simulink model "Simulation"  (R2019b)
settings: Solver=VariableStepAuto  StartTime=0.0  StopTime=tmax  RelTol=1e-3
values from neighbouring files (symbols this model uses):
  BPden = [1 alpha]    [RunSimulation.m]    (also in RunTest.m)
  BPnum = [0.3 alpha]    [RunSimulation.m]    (also in RunTest.m)
  c = 250    [RunSimulation.m]    (also in RunTest.m)
  efficiency = 0.95    [RunSimulation.m]
  Fb = -1*m    (= -90000)    [RunSimulation.m]
  l = 18    [RunSimulation.m]    (also in RunTest.m)
  m = 90000    [RunSimulation.m]
  p0 = 0    [RunSimulation.m]    (also in RunTest.m)
  Pres = 0/1000*[5.7/771 0 1.6]    [RunSimulation.m]    (also in RunTest.m)
  RBD = 5    [RunSimulation.m]    (also in RunTest.m)
  tl = .1    (= 0.1)    [RunSimulation.m]    (also in RunTest.m)
  trackgradient = 0    [RunSimulation.m]    (also in RunTest.m)
  trainpower = m    (= 90000)    [RunSimulation.m]
  v0 = 100/3.6    (= 27.7777777778)    [RunSimulation.m]
  VBD = 3.5    [RunSimulation.m]    (also in RunTest.m)
libraries: simulink x11
(part 2 of 5)

== system Simulation/Subsystem1/Wagon model1 ==
  note: $F=F_a-F_{res}$
  note: $s(t)=v_{0}\cdot t-{1 \over 2}\cdot a\cdot t^{2}$
  note: $F=m\cdot a$ $a={F \over m}$
  p_BP : Inport
  In1 : Inport  Port=2
  Abs : Abs
  Add : Sum
  Clock : Clock
  Dead Zone : DeadZone  LowerValue=-0.001  UpperValue=0.001  SaturateOnIntegerOverflow=on
  Divide : Product  Inputs=*/
  Gain : Gain  Gain=-1/(RBD-VBD)
  Gain1 : Gain  Gain=Fb
  Gain2 : Gain  Gain=v0
  Gain3 : Gain  Gain=0.5
  Gravity : Gain  Gain=9.81
  Math Function : Math  Operator=square  SignedPower=off  SaturateOnIntegerOverflow=on
  Product : Product
  Product1 : Product
  Rate Limiter : RateLimiter  RisingSlewLimit=1/tf  FallingSlewLimit=-1/tl  SampleTimeMode=inherited
  Saturation : Saturate  UpperLimit=1  LowerLimit=0
  Strahl formula : Polyval  Coefs=Pres
  Subtract : Sum
  Sum1 : Sum  Inputs=|+-
  Transfer Fcn : TransferFcn  Numerator=BPnum  Denominator=BPden
  Transport Delay : TransportDelay  DelayTime=l/c  InitialOutput=p0
  efficiency : Gain  Gain=efficiency
  filter out going backwards : Saturate  UpperLimit=inf  LowerLimit=0
  mass : Constant  Value=m
  track gradient : Bias  Bias=9.81*sin(trackgradient)
  v = v0 + a * t : Integrator  InitialCondition=v0
  Fres : Outport  VectorParamsAs1DForOutWhenUnconnected=off
  p_BP_out : Outport  Port=2  VectorParamsAs1DForOutWhenUnconnected=off
  "v " : Outport  Port=3
  ares : Outport  Port=4
  st : Outport  Port=5
  wires:
  Strahl formula/1 -> Gravity/1
  Abs/1 -> "v "/1, Strahl formula/1
  Gravity/1 -> Product/2
  Product/1 -> Sum1/2  "Fw"
  v = v0 + a * t/1 -> Abs/1  "v"
  mass/1 -> Product/1, Divide/2
  Divide/1 -> track gradient/1  "a"
  p_BP/1 -> Transport Delay/1, Dead Zone/1
  Gain/1 -> Saturation/1
  Gain1/1 -> efficiency/1
  Saturation/1 -> Rate Limiter/1
  Rate Limiter/1 -> Gain1/1
  Transfer Fcn/1 -> p_BP_out/1
  Transport Delay/1 -> Transfer Fcn/1
  efficiency/1 -> Sum1/1
  track gradient/1 -> ares/1, Product1/2, v = v0 + a * t/1  "ares"
  Clock/1 -> Math Function/1, Gain2/1
  Math Function/1 -> Product1/1
  Product1/1 -> Gain3/1
  Subtract/1 -> filter out going backwards/1
  Gain3/1 -> Subtract/1
  Gain2/1 -> Subtract/2
  filter out going backwards/1 -> st/1
  Dead Zone/1 -> Gain/1
  In1/1 -> Add/1  "Fa"
  Sum1/1 -> Add/2  "Fres"
  Add/1 -> Fres/1, Divide/1  "F"

== system Simulation/Subsystem1/Wagon model2 ==
  note: $F=F_a-F_{res}$
  note: $s(t)=v_{0}\cdot t-{1 \over 2}\cdot a\cdot t^{2}$
  note: $F=m\cdot a$ $a={F \over m}$
  p_BP : Inport
  In1 : Inport  Port=2
  Abs : Abs
  Add : Sum
  Clock : Clock
  Dead Zone : DeadZone  LowerValue=-0.001  UpperValue=0.001  SaturateOnIntegerOverflow=on
  Divide : Product  Inputs=*/
  Gain : Gain  Gain=-1/(RBD-VBD)
  Gain1 : Gain  Gain=Fb
  Gain2 : Gain  Gain=v0
  Gain3 : Gain  Gain=0.5
  Gravity : Gain  Gain=9.81
  Math Function : Math  Operator=square  SignedPower=off  SaturateOnIntegerOverflow=on
  Product : Product
  Product1 : Product
  Rate Limiter : RateLimiter  RisingSlewLimit=1/tf  FallingSlewLimit=-1/tl  SampleTimeMode=inherited
  Saturation : Saturate  UpperLimit=1  LowerLimit=0
  Strahl formula : Polyval  Coefs=Pres
  Subtract : Sum
  Sum1 : Sum  Inputs=|+-
  Transfer Fcn : TransferFcn  Numerator=BPnum  Denominator=BPden
  Transport Delay : TransportDelay  DelayTime=l/c  InitialOutput=p0
  efficiency : Gain  Gain=efficiency
  filter out going backwards : Saturate  UpperLimit=inf  LowerLimit=0
  mass : Constant  Value=m
  track gradient : Bias  Bias=9.81*sin(trackgradient)
  v = v0 + a * t : Integrator  InitialCondition=v0
  Fres : Outport  VectorParamsAs1DForOutWhenUnconnected=off
  p_BP_out : Outport  Port=2  VectorParamsAs1DForOutWhenUnconnected=off
  "v " : Outport  Port=3
  ares : Outport  Port=4
  st : Outport  Port=5
  wires:
  Strahl formula/1 -> Gravity/1
  Abs/1 -> "v "/1, Strahl formula/1
  Gravity/1 -> Product/2
  Product/1 -> Sum1/2  "Fw"
  v = v0 + a * t/1 -> Abs/1  "v"
  mass/1 -> Product/1, Divide/2
  Divide/1 -> track gradient/1  "a"
  p_BP/1 -> Transport Delay/1, Dead Zone/1
  Gain/1 -> Saturation/1
  Gain1/1 -> efficiency/1
  Saturation/1 -> Rate Limiter/1
  Rate Limiter/1 -> Gain1/1
  Transfer Fcn/1 -> p_BP_out/1
  Transport Delay/1 -> Transfer Fcn/1
  efficiency/1 -> Sum1/1
  track gradient/1 -> ares/1, Product1/2, v = v0 + a * t/1  "ares"
  Clock/1 -> Math Function/1, Gain2/1
  Math Function/1 -> Product1/1
  Product1/1 -> Gain3/1
  Subtract/1 -> filter out going backwards/1
  Gain3/1 -> Subtract/1
  Gain2/1 -> Subtract/2
  filter out going backwards/1 -> st/1
  Dead Zone/1 -> Gain/1
  In1/1 -> Add/1  "Fa"
  Sum1/1 -> Add/2  "Fres"
  Add/1 -> Fres/1, Divide/1  "F"

== system Simulation/Subsystem1/Wagon model3 ==
  note: $F=F_a-F_{res}$
  note: $s(t)=v_{0}\cdot t-{1 \over 2}\cdot a\cdot t^{2}$
  note: $F=m\cdot a$ $a={F \over m}$
  p_BP : Inport
  In1 : Inport  Port=2
  Abs : Abs
  Add : Sum
  Clock : Clock
  Dead Zone : DeadZone  LowerValue=-0.001  UpperValue=0.001  SaturateOnIntegerOverflow=on
  Divide : Product  Inputs=*/
  Gain : Gain  Gain=-1/(RBD-VBD)
  Gain1 : Gain  Gain=Fb
  Gain2 : Gain  Gain=v0
  Gain3 : Gain  Gain=0.5
  Gravity : Gain  Gain=9.81
  Math Function : Math  Operator=square  SignedPower=off  SaturateOnIntegerOverflow=on
  Product : Product
  Product1 : Product
  Rate Limiter : RateLimiter  RisingSlewLimit=1/tf  FallingSlewLimit=-1/tl  SampleTimeMode=inherited
  Saturation : Saturate  UpperLimit=1  LowerLimit=0
  Strahl formula : Polyval  Coefs=Pres
  Subtract : Sum
  Sum1 : Sum  Inputs=|+-
  Transfer Fcn : TransferFcn  Numerator=BPnum  Denominator=BPden
  Transport Delay : TransportDelay  DelayTime=l/c  InitialOutput=p0
  efficiency : Gain  Gain=efficiency
  filter out going backwards : Saturate  UpperLimit=inf  LowerLimit=0
  mass : Constant  Value=m
  track gradient : Bias  Bias=9.81*sin(trackgradient)
  v = v0 + a * t : Integrator  InitialCondition=v0
  Fres : Outport  VectorParamsAs1DForOutWhenUnconnected=off
  p_BP_out : Outport  Port=2  VectorParamsAs1DForOutWhenUnconnected=off
  "v " : Outport  Port=3
  ares : Outport  Port=4
  st : Outport  Port=5
  wires:
  Strahl formula/1 -> Gravity/1
  Abs/1 -> "v "/1, Strahl formula/1
  Gravity/1 -> Product/2
  Product/1 -> Sum1/2  "Fw"
  v = v0 + a * t/1 -> Abs/1  "v"
  mass/1 -> Product/1, Divide/2
  Divide/1 -> track gradient/1  "a"
  p_BP/1 -> Transport Delay/1, Dead Zone/1
  Gain/1 -> Saturation/1
  Gain1/1 -> efficiency/1
  Saturation/1 -> Rate Limiter/1
  Rate Limiter/1 -> Gain1/1
  Transfer Fcn/1 -> p_BP_out/1
  Transport Delay/1 -> Transfer Fcn/1
  efficiency/1 -> Sum1/1
  track gradient/1 -> ares/1, Product1/2, v = v0 + a * t/1  "ares"
  Clock/1 -> Math Function/1, Gain2/1
  Math Function/1 -> Product1/1
  Product1/1 -> Gain3/1
  Subtract/1 -> filter out going backwards/1
  Gain3/1 -> Subtract/1
  Gain2/1 -> Subtract/2
  filter out going backwards/1 -> st/1
  Dead Zone/1 -> Gain/1
  In1/1 -> Add/1  "Fa"
  Sum1/1 -> Add/2  "Fres"
  Add/1 -> Fres/1, Divide/1  "F"

== system Simulation/Subsystem1/Wagon model4 ==
  note: $F=F_a-F_{res}$
  note: $s(t)=v_{0}\cdot t-{1 \over 2}\cdot a\cdot t^{2}$
  note: $F=m\cdot a$ $a={F \over m}$
  p_BP : Inport
  In1 : Inport  Port=2
  Abs : Abs
  Add : Sum
  Clock : Clock
  Dead Zone : DeadZone  LowerValue=-0.001  UpperValue=0.001  SaturateOnIntegerOverflow=on
  Divide : Product  Inputs=*/
  Gain : Gain  Gain=-1/(RBD-VBD)
  Gain1 : Gain  Gain=Fb
  Gain2 : Gain  Gain=v0
  Gain3 : Gain  Gain=0.5
  Gravity : Gain  Gain=9.81
  Math Function : Math  Operator=square  SignedPower=off  SaturateOnIntegerOverflow=on
  Product : Product
  Product1 : Product
  Rate Limiter : RateLimiter  RisingSlewLimit=1/tf  FallingSlewLimit=-1/tl  SampleTimeMode=inherited
  Saturation : Saturate  UpperLimit=1  LowerLimit=0
  Strahl formula : Polyval  Coefs=Pres
  Subtract : Sum
  Sum1 : Sum  Inputs=|+-
  Transfer Fcn : TransferFcn  Numerator=BPnum  Denominator=BPden
  Transport Delay : TransportDelay  DelayTime=l/c  InitialOutput=p0
  efficiency : Gain  Gain=efficiency
  filter out going backwards : Saturate  UpperLimit=inf  LowerLimit=0
  mass : Constant  Value=m
  track gradient : Bias  Bias=9.81*sin(trackgradient)
  v = v0 + a * t : Integrator  InitialCondition=v0
  Fres : Outport  VectorParamsAs1DForOutWhenUnconnected=off
  p_BP_out : Outport  Port=2  VectorParamsAs1DForOutWhenUnconnected=off
  "v " : Outport  Port=3
  ares : Outport  Port=4
  st : Outport  Port=5
  wires:
  Strahl formula/1 -> Gravity/1
  Abs/1 -> "v "/1, Strahl formula/1
  Gravity/1 -> Product/2
  Product/1 -> Sum1/2  "Fw"
  v = v0 + a * t/1 -> Abs/1  "v"
  mass/1 -> Product/1, Divide/2
  Divide/1 -> track gradient/1  "a"
  p_BP/1 -> Transport Delay/1, Dead Zone/1
  Gain/1 -> Saturation/1
  Gain1/1 -> efficiency/1
  Saturation/1 -> Rate Limiter/1
  Rate Limiter/1 -> Gain1/1
  Transfer Fcn/1 -> p_BP_out/1
  Transport Delay/1 -> Transfer Fcn/1
  efficiency/1 -> Sum1/1
  track gradient/1 -> ares/1, Product1/2, v = v0 + a * t/1  "ares"
  Clock/1 -> Math Function/1, Gain2/1
  Math Function/1 -> Product1/1
  Product1/1 -> Gain3/1
  Subtract/1 -> filter out going backwards/1
  Gain3/1 -> Subtract/1
  Gain2/1 -> Subtract/2
  filter out going backwards/1 -> st/1
  Dead Zone/1 -> Gain/1
  In1/1 -> Add/1  "Fa"
  Sum1/1 -> Add/2  "Fres"
  Add/1 -> Fres/1, Divide/1  "F"

== system Simulation/Subsystem10/Wagon model ==
  note: F = m * a
      | a = F / m
  p_BP : Inport
  Abs : Abs
  Constant : Constant  Value=m
  Divide : Product  Inputs=*/
  Gain : Gain  Gain=-1/(RBD-VBD)
  Gain1 : Gain  Gain=Fb
  Gravity : Gain  Gain=9.81
  Product : Product
  Rate Limiter : RateLimiter  RisingSlewLimit=1/tf  FallingSlewLimit=-1/tl  SampleTimeMode=inherited
  Saturation : Saturate  UpperLimit=1  LowerLimit=0
  Strahl formula : Polyval  Coefs=Pres
  Sum1 : Sum  Inputs=|+-
  Transfer Fcn : TransferFcn  Numerator=BPnum  Denominator=BPden
  Transport Delay : TransportDelay  DelayTime=l/c  InitialOutput=p0
  filter out negative velocity : Saturate  UpperLimit=inf  LowerLimit=0
  v = v0 + a * t : Integrator  InitialCondition=v0
  Fres : Outport  VectorParamsAs1DForOutWhenUnconnected=off
  p_BP_out : Outport  Port=2  VectorParamsAs1DForOutWhenUnconnected=off
  "v " : Outport  Port=3
  wires:
  Sum1/1 -> Fres/1, Divide/1  "Fres"
  Strahl formula/1 -> Gravity/1
  Abs/1 -> Strahl formula/1
  Gravity/1 -> Product/2
  Product/1 -> Sum1/2  "Fw"
  v = v0 + a * t/1 -> filter out negative velocity/1, Abs/1  "v"
  Constant/1 -> Product/1, Divide/2
  Divide/1 -> v = v0 + a * t/1  "a"
  p_BP/1 -> Transport Delay/1, Gain/1
  Gain/1 -> Saturation/1
  Gain1/1 -> Sum1/1
  Saturation/1 -> Rate Limiter/1
  Rate Limiter/1 -> Gain1/1
  Transfer Fcn/1 -> p_BP_out/1
  Transport Delay/1 -> Transfer Fcn/1
  filter out negative velocity/1 -> "v "/1

== system Simulation/Subsystem10/Wagon model1 ==
  p_BP : Inport
  Abs : Abs
  Constant : Constant  Value=m
  Divide : Product  Inputs=*/
  Gain : Gain  Gain=-1/(RBD-VBD)
  Gain1 : Gain  Gain=Fb
  Gravity : Gain  Gain=9.81
  Integrator : Integrator  InitialCondition=v0
  Product : Product
  Rate Limiter : RateLimiter  RisingSlewLimit=1/tf  FallingSlewLimit=-1/tl  SampleTimeMode=inherited
  Saturation : Saturate  UpperLimit=1  LowerLimit=0
  Strahl formula : Polyval  Coefs=Pres
  Sum1 : Sum  Inputs=|+-
  Transfer Fcn : TransferFcn  Numerator=BPnum  Denominator=BPden
  Transport Delay : TransportDelay  DelayTime=l/c  InitialOutput=p0
  filter out negative velocity : Saturate  UpperLimit=inf  LowerLimit=0
  Fres : Outport  VectorParamsAs1DForOutWhenUnconnected=off
  p_BP_out : Outport  Port=2  VectorParamsAs1DForOutWhenUnconnected=off
  "v " : Outport  Port=3
  wires:
  Sum1/1 -> Fres/1, Divide/1  "Fres"
  Strahl formula/1 -> Gravity/1
  Abs/1 -> Strahl formula/1
  Gravity/1 -> Product/2
  Product/1 -> Sum1/2  "Fw"
  Integrator/1 -> filter out negative velocity/1, Abs/1  "v"
  Constant/1 -> Product/1, Divide/2
  Divide/1 -> Integrator/1  "a"
  p_BP/1 -> Gain/1, Transport Delay/1
  Gain/1 -> Saturation/1
  Gain1/1 -> Sum1/1
  Saturation/1 -> Rate Limiter/1
  Rate Limiter/1 -> Gain1/1
  Transport Delay/1 -> Transfer Fcn/1
  Transfer Fcn/1 -> p_BP_out/1
  filter out negative velocity/1 -> "v "/1

== system Simulation/Subsystem10/Wagon model2 ==
  p_BP : Inport
  Abs : Abs
  Constant : Constant  Value=m
  Divide : Product  Inputs=*/
  Gain : Gain  Gain=-1/(RBD-VBD)
  Gain1 : Gain  Gain=Fb
  Gravity : Gain  Gain=9.81
  Integrator : Integrator  InitialCondition=v0
  Product : Product
  Rate Limiter : RateLimiter  RisingSlewLimit=1/tf  FallingSlewLimit=-1/tl  SampleTimeMode=inherited
  Saturation : Saturate  UpperLimit=1  LowerLimit=0
  Strahl formula : Polyval  Coefs=Pres
  Sum1 : Sum  Inputs=|+-
  Transfer Fcn : TransferFcn  Numerator=BPnum  Denominator=BPden
  Transport Delay : TransportDelay  DelayTime=l/c  InitialOutput=p0
  filter out negative velocity : Saturate  UpperLimit=inf  LowerLimit=0
  Fres : Outport  VectorParamsAs1DForOutWhenUnconnected=off
  p_BP_out : Outport  Port=2  VectorParamsAs1DForOutWhenUnconnected=off
  "v " : Outport  Port=3
  wires:
  Sum1/1 -> Fres/1, Divide/1  "Fres"
  Strahl formula/1 -> Gravity/1
  Abs/1 -> Strahl formula/1
  Gravity/1 -> Product/2
  Product/1 -> Sum1/2  "Fw"
  Constant/1 -> Product/1, Divide/2
  Divide/1 -> Integrator/1  "a"
  p_BP/1 -> Gain/1, Transport Delay/1
  Gain/1 -> Saturation/1
  Gain1/1 -> Sum1/1
  Saturation/1 -> Rate Limiter/1
  Rate Limiter/1 -> Gain1/1
  Transport Delay/1 -> Transfer Fcn/1
  Transfer Fcn/1 -> p_BP_out/1
  Integrator/1 -> filter out negative velocity/1, Abs/1  "v"
  filter out negative velocity/1 -> "v "/1

== system Simulation/Subsystem10/Wagon model3 ==
  p_BP : Inport
  Abs : Abs
  Constant : Constant  Value=m
  Divide : Product  Inputs=*/
  Gain : Gain  Gain=-1/(RBD-VBD)
  Gain1 : Gain  Gain=Fb
  Gravity : Gain  Gain=9.81
  Integrator : Integrator  InitialCondition=v0
  Product : Product
  Rate Limiter : RateLimiter  RisingSlewLimit=1/tf  FallingSlewLimit=-1/tl  SampleTimeMode=inherited
  Saturation : Saturate  UpperLimit=1  LowerLimit=0
  Strahl formula : Polyval  Coefs=Pres
  Sum1 : Sum  Inputs=|+-
  Transfer Fcn : TransferFcn  Numerator=BPnum  Denominator=BPden
  Transport Delay : TransportDelay  DelayTime=l/c  InitialOutput=p0
  filter out negative velocity : Saturate  UpperLimit=inf  LowerLimit=0
  Fres : Outport  VectorParamsAs1DForOutWhenUnconnected=off
  p_BP_out : Outport  Port=2  VectorParamsAs1DForOutWhenUnconnected=off
  "v " : Outport  Port=3
  wires:
  Sum1/1 -> Fres/1, Divide/1  "Fres"
  Strahl formula/1 -> Gravity/1
  Abs/1 -> Strahl formula/1
  Gravity/1 -> Product/2
  Product/1 -> Sum1/2  "Fw"
  Constant/1 -> Product/1, Divide/2
  Divide/1 -> Integrator/1  "a"
  p_BP/1 -> Gain/1, Transport Delay/1
  Gain/1 -> Saturation/1
  Gain1/1 -> Sum1/1
  Saturation/1 -> Rate Limiter/1
  Rate Limiter/1 -> Gain1/1
  Transport Delay/1 -> Transfer Fcn/1
  Transfer Fcn/1 -> p_BP_out/1
  Integrator/1 -> Abs/1, filter out negative velocity/1  "v"
  filter out negative velocity/1 -> "v "/1

== system Simulation/Subsystem10/Wagon model4 ==
  p_BP : Inport
  Abs : Abs
  Constant : Constant  Value=m
  Divide : Product  Inputs=*/
  Gain : Gain  Gain=-1/(RBD-VBD)
  Gain1 : Gain  Gain=Fb
  Gravity : Gain  Gain=9.81
  Integrator : Integrator  InitialCondition=v0
  Product : Product
  Rate Limiter : RateLimiter  RisingSlewLimit=1/tf  FallingSlewLimit=-1/tl  SampleTimeMode=inherited
  Saturation : Saturate  UpperLimit=1  LowerLimit=0
  Strahl formula : Polyval  Coefs=Pres
  Sum1 : Sum  Inputs=|+-
  Transfer Fcn : TransferFcn  Numerator=BPnum  Denominator=BPden
  Transport Delay : TransportDelay  DelayTime=l/c  InitialOutput=p0
  filter out negative velocity : Saturate  UpperLimit=inf  LowerLimit=0
  Fres : Outport  VectorParamsAs1DForOutWhenUnconnected=off
  p_BP_out : Outport  Port=2  VectorParamsAs1DForOutWhenUnconnected=off
  "v " : Outport  Port=3
  wires:
  Sum1/1 -> Fres/1, Divide/1  "Fres"
  Strahl formula/1 -> Gravity/1
  Abs/1 -> Strahl formula/1
  Gravity/1 -> Product/2
  Product/1 -> Sum1/2  "Fw"
  Integrator/1 -> filter out negative velocity/1, Abs/1  "v"
  Constant/1 -> Product/1, Divide/2
  Divide/1 -> Integrator/1  "a"
  p_BP/1 -> Gain/1, Transport Delay/1
  Gain/1 -> Saturation/1
  Gain1/1 -> Sum1/1
  Saturation/1 -> Rate Limiter/1
  Rate Limiter/1 -> Gain1/1
  Transfer Fcn/1 -> p_BP_out/1
  Transport Delay/1 -> Transfer Fcn/1
  filter out negative velocity/1 -> "v "/1

== system Simulation/Subsystem11/Wagon model ==
  note: F = m * a
      | a = F / m
  p_BP : Inport
  Abs : Abs
  Constant : Constant  Value=m
  Divide : Product  Inputs=*/
  Gain : Gain  Gain=-1/(RBD-VBD)
  Gain1 : Gain  Gain=Fb
  Gravity : Gain  Gain=9.81
  Product : Product
  Rate Limiter : RateLimiter  RisingSlewLimit=1/tf  FallingSlewLimit=-1/tl  SampleTimeMode=inherited
  Saturation : Saturate  UpperLimit=1  LowerLimit=0
  Strahl formula : Polyval  Coefs=Pres
  Sum1 : Sum  Inputs=|+-
  Transfer Fcn : TransferFcn  Numerator=BPnum  Denominator=BPden
  Transport Delay : TransportDelay  DelayTime=l/c  InitialOutput=p0
  filter out negative velocity : Saturate  UpperLimit=inf  LowerLimit=0
  v = v0 + a * t : Integrator  InitialCondition=v0
  Fres : Outport  VectorParamsAs1DForOutWhenUnconnected=off
  p_BP_out : Outport  Port=2  VectorParamsAs1DForOutWhenUnconnected=off
  "v " : Outport  Port=3
  wires:
  Sum1/1 -> Fres/1, Divide/1  "Fres"
  Strahl formula/1 -> Gravity/1
  Abs/1 -> Strahl formula/1
  Gravity/1 -> Product/2
  Product/1 -> Sum1/2  "Fw"
  v = v0 + a * t/1 -> filter out negative velocity/1, Abs/1  "v"
  Constant/1 -> Product/1, Divide/2
  Divide/1 -> v = v0 + a * t/1  "a"
  p_BP/1 -> Transport Delay/1, Gain/1
  Gain/1 -> Saturation/1
  Gain1/1 -> Sum1/1
  Saturation/1 -> Rate Limiter/1
  Rate Limiter/1 -> Gain1/1
  Transfer Fcn/1 -> p_BP_out/1
  Transport Delay/1 -> Transfer Fcn/1
  filter out negative velocity/1 -> "v "/1

== system Simulation/Subsystem11/Wagon model1 ==
  p_BP : Inport
  Abs : Abs
  Constant : Constant  Value=m
  Divide : Product  Inputs=*/
  Gain : Gain  Gain=-1/(RBD-VBD)
  Gain1 : Gain  Gain=Fb
  Gravity : Gain  Gain=9.81
  Integrator : Integrator  InitialCondition=v0
  Product : Product
  Rate Limiter : RateLimiter  RisingSlewLimit=1/tf  FallingSlewLimit=-1/tl  SampleTimeMode=inherited
  Saturation : Saturate  UpperLimit=1  LowerLimit=0
  Strahl formula : Polyval  Coefs=Pres
  Sum1 : Sum  Inputs=|+-
  Transfer Fcn : TransferFcn  Numerator=BPnum  Denominator=BPden
  Transport Delay : TransportDelay  DelayTime=l/c  InitialOutput=p0
  filter out negative velocity : Saturate  UpperLimit=inf  LowerLimit=0
  Fres : Outport  VectorParamsAs1DForOutWhenUnconnected=off
  p_BP_out : Outport  Port=2  VectorParamsAs1DForOutWhenUnconnected=off
  "v " : Outport  Port=3
  wires:
  Sum1/1 -> Fres/1, Divide/1  "Fres"
  Strahl formula/1 -> Gravity/1
  Abs/1 -> Strahl formula/1
  Gravity/1 -> Product/2
  Product/1 -> Sum1/2  "Fw"
  Integrator/1 -> filter out negative velocity/1, Abs/1  "v"
  Constant/1 -> Product/1, Divide/2
  Divide/1 -> Integrator/1  "a"
  p_BP/1 -> Gain/1, Transport Delay/1
  Gain/1 -> Saturation/1
  Gain1/1 -> Sum1/1
  Saturation/1 -> Rate Limiter/1
  Rate Limiter/1 -> Gain1/1
  Transport Delay/1 -> Transfer Fcn/1
  Transfer Fcn/1 -> p_BP_out/1
  filter out negative velocity/1 -> "v "/1

== system Simulation/Subsystem11/Wagon model2 ==
  p_BP : Inport
  Abs : Abs
  Constant : Constant  Value=m
  Divide : Product  Inputs=*/
  Gain : Gain  Gain=-1/(RBD-VBD)
  Gain1 : Gain  Gain=Fb
  Gravity : Gain  Gain=9.81
  Integrator : Integrator  InitialCondition=v0
  Product : Product
  Rate Limiter : RateLimiter  RisingSlewLimit=1/tf  FallingSlewLimit=-1/tl  SampleTimeMode=inherited
  Saturation : Saturate  UpperLimit=1  LowerLimit=0
  Strahl formula : Polyval  Coefs=Pres
  Sum1 : Sum  Inputs=|+-
  Transfer Fcn : TransferFcn  Numerator=BPnum  Denominator=BPden
  Transport Delay : TransportDelay  DelayTime=l/c  InitialOutput=p0
  filter out negative velocity : Saturate  UpperLimit=inf  LowerLimit=0
  Fres : Outport  VectorParamsAs1DForOutWhenUnconnected=off
  p_BP_out : Outport  Port=2  VectorParamsAs1DForOutWhenUnconnected=off
  "v " : Outport  Port=3
  wires:
  Sum1/1 -> Fres/1, Divide/1  "Fres"
  Strahl formula/1 -> Gravity/1
  Abs/1 -> Strahl formula/1
  Gravity/1 -> Product/2
  Product/1 -> Sum1/2  "Fw"
  Constant/1 -> Product/1, Divide/2
  Divide/1 -> Integrator/1  "a"
  p_BP/1 -> Gain/1, Transport Delay/1
  Gain/1 -> Saturation/1
  Gain1/1 -> Sum1/1
  Saturation/1 -> Rate Limiter/1
  Rate Limiter/1 -> Gain1/1
  Transport Delay/1 -> Transfer Fcn/1
  Transfer Fcn/1 -> p_BP_out/1
  Integrator/1 -> filter out negative velocity/1, Abs/1  "v"
  filter out negative velocity/1 -> "v "/1

== system Simulation/Subsystem11/Wagon model3 ==
  p_BP : Inport
  Abs : Abs
  Constant : Constant  Value=m
  Divide : Product  Inputs=*/
  Gain : Gain  Gain=-1/(RBD-VBD)
  Gain1 : Gain  Gain=Fb
  Gravity : Gain  Gain=9.81
  Integrator : Integrator  InitialCondition=v0
  Product : Product
  Rate Limiter : RateLimiter  RisingSlewLimit=1/tf  FallingSlewLimit=-1/tl  SampleTimeMode=inherited
  Saturation : Saturate  UpperLimit=1  LowerLimit=0
  Strahl formula : Polyval  Coefs=Pres
  Sum1 : Sum  Inputs=|+-
  Transfer Fcn : TransferFcn  Numerator=BPnum  Denominator=BPden
  Transport Delay : TransportDelay  DelayTime=l/c  InitialOutput=p0
  filter out negative velocity : Saturate  UpperLimit=inf  LowerLimit=0
  Fres : Outport  VectorParamsAs1DForOutWhenUnconnected=off
  p_BP_out : Outport  Port=2  VectorParamsAs1DForOutWhenUnconnected=off
  "v " : Outport  Port=3
  wires:
  Sum1/1 -> Fres/1, Divide/1  "Fres"
  Strahl formula/1 -> Gravity/1
  Abs/1 -> Strahl formula/1
  Gravity/1 -> Product/2
  Product/1 -> Sum1/2  "Fw"
  Constant/1 -> Product/1, Divide/2
  Divide/1 -> Integrator/1  "a"
  p_BP/1 -> Gain/1, Transport Delay/1
  Gain/1 -> Saturation/1
  Gain1/1 -> Sum1/1
  Saturation/1 -> Rate Limiter/1
  Rate Limiter/1 -> Gain1/1
  Transport Delay/1 -> Transfer Fcn/1
  Transfer Fcn/1 -> p_BP_out/1
  Integrator/1 -> Abs/1, filter out negative velocity/1  "v"
  filter out negative velocity/1 -> "v "/1

== system Simulation/Subsystem11/Wagon model4 ==
  p_BP : Inport
  Abs : Abs
  Constant : Constant  Value=m
  Divide : Product  Inputs=*/
  Gain : Gain  Gain=-1/(RBD-VBD)
  Gain1 : Gain  Gain=Fb
  Gravity : Gain  Gain=9.81
  Integrator : Integrator  InitialCondition=v0
  Product : Product
  Rate Limiter : RateLimiter  RisingSlewLimit=1/tf  FallingSlewLimit=-1/tl  SampleTimeMode=inherited
  Saturation : Saturate  UpperLimit=1  LowerLimit=0
  Strahl formula : Polyval  Coefs=Pres
  Sum1 : Sum  Inputs=|+-
  Transfer Fcn : TransferFcn  Numerator=BPnum  Denominator=BPden
  Transport Delay : TransportDelay  DelayTime=l/c  InitialOutput=p0
  filter out negative velocity : Saturate  UpperLimit=inf  LowerLimit=0
  Fres : Outport  VectorParamsAs1DForOutWhenUnconnected=off
  p_BP_out : Outport  Port=2  VectorParamsAs1DForOutWhenUnconnected=off
  "v " : Outport  Port=3
  wires:
  Sum1/1 -> Fres/1, Divide/1  "Fres"
  Strahl formula/1 -> Gravity/1
  Abs/1 -> Strahl formula/1
  Gravity/1 -> Product/2
  Product/1 -> Sum1/2  "Fw"
  Integrator/1 -> filter out negative velocity/1, Abs/1  "v"
  Constant/1 -> Product/1, Divide/2
  Divide/1 -> Integrator/1  "a"
  p_BP/1 -> Gain/1, Transport Delay/1
  Gain/1 -> Saturation/1
  Gain1/1 -> Sum1/1
  Saturation/1 -> Rate Limiter/1
  Rate Limiter/1 -> Gain1/1
  Transfer Fcn/1 -> p_BP_out/1
  Transport Delay/1 -> Transfer Fcn/1
  filter out negative velocity/1 -> "v "/1

== system Simulation/Subsystem12/Wagon model ==
  note: F = m * a
      | a = F / m
  p_BP : Inport
  Abs : Abs
  Constant : Constant  Value=m
  Divide : Product  Inputs=*/
  Gain : Gain  Gain=-1/(RBD-VBD)
  Gain1 : Gain  Gain=Fb
  Gravity : Gain  Gain=9.81
  Product : Product
  Rate Limiter : RateLimiter  RisingSlewLimit=1/tf  FallingSlewLimit=-1/tl  SampleTimeMode=inherited
  Saturation : Saturate  UpperLimit=1  LowerLimit=0
  Strahl formula : Polyval  Coefs=Pres
  Sum1 : Sum  Inputs=|+-
  Transfer Fcn : TransferFcn  Numerator=BPnum  Denominator=BPden
  Transport Delay : TransportDelay  DelayTime=l/c  InitialOutput=p0
  filter out negative velocity : Saturate  UpperLimit=inf  LowerLimit=0
  v = v0 + a * t : Integrator  InitialCondition=v0
  Fres : Outport  VectorParamsAs1DForOutWhenUnconnected=off
  p_BP_out : Outport  Port=2  VectorParamsAs1DForOutWhenUnconnected=off
  "v " : Outport  Port=3
  wires:
  Sum1/1 -> Fres/1, Divide/1  "Fres"
  Strahl formula/1 -> Gravity/1
  Abs/1 -> Strahl formula/1
  Gravity/1 -> Product/2
  Product/1 -> Sum1/2  "Fw"
  v = v0 + a * t/1 -> filter out negative velocity/1, Abs/1  "v"
  Constant/1 -> Product/1, Divide/2
  Divide/1 -> v = v0 + a * t/1  "a"
  p_BP/1 -> Transport Delay/1, Gain/1
  Gain/1 -> Saturation/1
  Gain1/1 -> Sum1/1
  Saturation/1 -> Rate Limiter/1
  Rate Limiter/1 -> Gain1/1
  Transfer Fcn/1 -> p_BP_out/1
  Transport Delay/1 -> Transfer Fcn/1
  filter out negative velocity/1 -> "v "/1

== system Simulation/Subsystem12/Wagon model1 ==
  p_BP : Inport
  Abs : Abs
  Constant : Constant  Value=m
  Divide : Product  Inputs=*/
  Gain : Gain  Gain=-1/(RBD-VBD)
  Gain1 : Gain  Gain=Fb
  Gravity : Gain  Gain=9.81
  Integrator : Integrator  InitialCondition=v0
  Product : Product
  Rate Limiter : RateLimiter  RisingSlewLimit=1/tf  FallingSlewLimit=-1/tl  SampleTimeMode=inherited
  Saturation : Saturate  UpperLimit=1  LowerLimit=0
  Strahl formula : Polyval  Coefs=Pres
  Sum1 : Sum  Inputs=|+-
  Transfer Fcn : TransferFcn  Numerator=BPnum  Denominator=BPden
  Transport Delay : TransportDelay  DelayTime=l/c  InitialOutput=p0
  filter out negative velocity : Saturate  UpperLimit=inf  LowerLimit=0
  Fres : Outport  VectorParamsAs1DForOutWhenUnconnected=off
  p_BP_out : Outport  Port=2  VectorParamsAs1DForOutWhenUnconnected=off
  "v " : Outport  Port=3
  wires:
  Sum1/1 -> Fres/1, Divide/1  "Fres"
  Strahl formula/1 -> Gravity/1
  Abs/1 -> Strahl formula/1
  Gravity/1 -> Product/2
  Product/1 -> Sum1/2  "Fw"
  Integrator/1 -> filter out negative velocity/1, Abs/1  "v"
  Constant/1 -> Product/1, Divide/2
  Divide/1 -> Integrator/1  "a"
  p_BP/1 -> Gain/1, Transport Delay/1
  Gain/1 -> Saturation/1
  Gain1/1 -> Sum1/1
  Saturation/1 -> Rate Limiter/1
  Rate Limiter/1 -> Gain1/1
  Transport Delay/1 -> Transfer Fcn/1
  Transfer Fcn/1 -> p_BP_out/1
  filter out negative velocity/1 -> "v "/1

== system Simulation/Subsystem12/Wagon model2 ==
  p_BP : Inport
  Abs : Abs
  Constant : Constant  Value=m
  Divide : Product  Inputs=*/
  Gain : Gain  Gain=-1/(RBD-VBD)
  Gain1 : Gain  Gain=Fb
  Gravity : Gain  Gain=9.81
  Integrator : Integrator  InitialCondition=v0
  Product : Product
  Rate Limiter : RateLimiter  RisingSlewLimit=1/tf  FallingSlewLimit=-1/tl  SampleTimeMode=inherited
  Saturation : Saturate  UpperLimit=1  LowerLimit=0
  Strahl formula : Polyval  Coefs=Pres
  Sum1 : Sum  Inputs=|+-
  Transfer Fcn : TransferFcn  Numerator=BPnum  Denominator=BPden
  Transport Delay : TransportDelay  DelayTime=l/c  InitialOutput=p0
  filter out negative velocity : Saturate  UpperLimit=inf  LowerLimit=0
  Fres : Outport  VectorParamsAs1DForOutWhenUnconnected=off
  p_BP_out : Outport  Port=2  VectorParamsAs1DForOutWhenUnconnected=off
  "v " : Outport  Port=3
  wires:
  Sum1/1 -> Fres/1, Divide/1  "Fres"
  Strahl formula/1 -> Gravity/1
  Abs/1 -> Strahl formula/1
  Gravity/1 -> Product/2
  Product/1 -> Sum1/2  "Fw"
  Constant/1 -> Product/1, Divide/2
  Divide/1 -> Integrator/1  "a"
  p_BP/1 -> Gain/1, Transport Delay/1
  Gain/1 -> Saturation/1
  Gain1/1 -> Sum1/1
  Saturation/1 -> Rate Limiter/1
  Rate Limiter/1 -> Gain1/1
  Transport Delay/1 -> Transfer Fcn/1
  Transfer Fcn/1 -> p_BP_out/1
  Integrator/1 -> filter out negative velocity/1, Abs/1  "v"
  filter out negative velocity/1 -> "v "/1

== system Simulation/Subsystem12/Wagon model3 ==
  p_BP : Inport
  Abs : Abs
  Constant : Constant  Value=m
  Divide : Product  Inputs=*/
  Gain : Gain  Gain=-1/(RBD-VBD)
  Gain1 : Gain  Gain=Fb
  Gravity : Gain  Gain=9.81
  Integrator : Integrator  InitialCondition=v0
  Product : Product
  Rate Limiter : RateLimiter  RisingSlewLimit=1/tf  FallingSlewLimit=-1/tl  SampleTimeMode=inherited
  Saturation : Saturate  UpperLimit=1  LowerLimit=0
  Strahl formula : Polyval  Coefs=Pres
  Sum1 : Sum  Inputs=|+-
  Transfer Fcn : TransferFcn  Numerator=BPnum  Denominator=BPden
  Transport Delay : TransportDelay  DelayTime=l/c  InitialOutput=p0
  filter out negative velocity : Saturate  UpperLimit=inf  LowerLimit=0
  Fres : Outport  VectorParamsAs1DForOutWhenUnconnected=off
  p_BP_out : Outport  Port=2  VectorParamsAs1DForOutWhenUnconnected=off
  "v " : Outport  Port=3
  wires:
  Sum1/1 -> Fres/1, Divide/1  "Fres"
  Strahl formula/1 -> Gravity/1
  Abs/1 -> Strahl formula/1
  Gravity/1 -> Product/2
  Product/1 -> Sum1/2  "Fw"
  Constant/1 -> Product/1, Divide/2
  Divide/1 -> Integrator/1  "a"
  p_BP/1 -> Gain/1, Transport Delay/1
  Gain/1 -> Saturation/1
  Gain1/1 -> Sum1/1
  Saturation/1 -> Rate Limiter/1
  Rate Limiter/1 -> Gain1/1
  Transport Delay/1 -> Transfer Fcn/1
  Transfer Fcn/1 -> p_BP_out/1
  Integrator/1 -> Abs/1, filter out negative velocity/1  "v"
  filter out negative velocity/1 -> "v "/1

== system Simulation/Subsystem12/Wagon model4 ==
  p_BP : Inport
  Abs : Abs
  Constant : Constant  Value=m
  Divide : Product  Inputs=*/
  Gain : Gain  Gain=-1/(RBD-VBD)
  Gain1 : Gain  Gain=Fb
  Gravity : Gain  Gain=9.81
  Integrator : Integrator  InitialCondition=v0
  Product : Product
  Rate Limiter : RateLimiter  RisingSlewLimit=1/tf  FallingSlewLimit=-1/tl  SampleTimeMode=inherited
  Saturation : Saturate  UpperLimit=1  LowerLimit=0
  Strahl formula : Polyval  Coefs=Pres
  Sum1 : Sum  Inputs=|+-
  Transfer Fcn : TransferFcn  Numerator=BPnum  Denominator=BPden
  Transport Delay : TransportDelay  DelayTime=l/c  InitialOutput=p0
  filter out negative velocity : Saturate  UpperLimit=inf  LowerLimit=0
  Fres : Outport  VectorParamsAs1DForOutWhenUnconnected=off
  p_BP_out : Outport  Port=2  VectorParamsAs1DForOutWhenUnconnected=off
  "v " : Outport  Port=3
  wires:
  Sum1/1 -> Fres/1, Divide/1  "Fres"
  Strahl formula/1 -> Gravity/1
  Abs/1 -> Strahl formula/1
  Gravity/1 -> Product/2
  Product/1 -> Sum1/2  "Fw"
  Integrator/1 -> filter out negative velocity/1, Abs/1  "v"
  Constant/1 -> Product/1, Divide/2
  Divide/1 -> Integrator/1  "a"
  p_BP/1 -> Gain/1, Transport Delay/1
  Gain/1 -> Saturation/1
  Gain1/1 -> Sum1/1
  Saturation/1 -> Rate Limiter/1
  Rate Limiter/1 -> Gain1/1
  Transfer Fcn/1 -> p_BP_out/1
  Transport Delay/1 -> Transfer Fcn/1
  filter out negative velocity/1 -> "v "/1

== system Simulation/Subsystem13/Wagon model ==
  note: F = m * a
      | a = F / m
  p_BP : Inport
  Abs : Abs
  Constant : Constant  Value=m
  Divide : Product  Inputs=*/
  Gain : Gain  Gain=-1/(RBD-VBD)
  Gain1 : Gain  Gain=Fb
  Gravity : Gain  Gain=9.81
  Product : Product
  Rate Limiter : RateLimiter  RisingSlewLimit=1/tf  FallingSlewLimit=-1/tl  SampleTimeMode=inherited
  Saturation : Saturate  UpperLimit=1  LowerLimit=0
  Strahl formula : Polyval  Coefs=Pres
  Sum1 : Sum  Inputs=|+-
  Transfer Fcn : TransferFcn  Numerator=BPnum  Denominator=BPden
  Transport Delay : TransportDelay  DelayTime=l/c  InitialOutput=p0
  filter out negative velocity : Saturate  UpperLimit=inf  LowerLimit=0
  v = v0 + a * t : Integrator  InitialCondition=v0
  Fres : Outport  VectorParamsAs1DForOutWhenUnconnected=off
  p_BP_out : Outport  Port=2  VectorParamsAs1DForOutWhenUnconnected=off
  "v " : Outport  Port=3
  wires:
  Sum1/1 -> Fres/1, Divide/1  "Fres"
  Strahl formula/1 -> Gravity/1
  Abs/1 -> Strahl formula/1
  Gravity/1 -> Product/2
  Product/1 -> Sum1/2  "Fw"
  v = v0 + a * t/1 -> filter out negative velocity/1, Abs/1  "v"
  Constant/1 -> Product/1, Divide/2
  Divide/1 -> v = v0 + a * t/1  "a"
  p_BP/1 -> Transport Delay/1, Gain/1
  Gain/1 -> Saturation/1
  Gain1/1 -> Sum1/1
  Saturation/1 -> Rate Limiter/1
  Rate Limiter/1 -> Gain1/1
  Transfer Fcn/1 -> p_BP_out/1
  Transport Delay/1 -> Transfer Fcn/1
  filter out negative velocity/1 -> "v "/1

== system Simulation/Subsystem13/Wagon model1 ==
  p_BP : Inport
  Abs : Abs
  Constant : Constant  Value=m
  Divide : Product  Inputs=*/
  Gain : Gain  Gain=-1/(RBD-VBD)
  Gain1 : Gain  Gain=Fb
  Gravity : Gain  Gain=9.81
  Integrator : Integrator  InitialCondition=v0
  Product : Product
  Rate Limiter : RateLimiter  RisingSlewLimit=1/tf  FallingSlewLimit=-1/tl  SampleTimeMode=inherited
  Saturation : Saturate  UpperLimit=1  LowerLimit=0
  Strahl formula : Polyval  Coefs=Pres
  Sum1 : Sum  Inputs=|+-
  Transfer Fcn : TransferFcn  Numerator=BPnum  Denominator=BPden
  Transport Delay : TransportDelay  DelayTime=l/c  InitialOutput=p0
  filter out negative velocity : Saturate  UpperLimit=inf  LowerLimit=0
  Fres : Outport  VectorParamsAs1DForOutWhenUnconnected=off
  p_BP_out : Outport  Port=2  VectorParamsAs1DForOutWhenUnconnected=off
  "v " : Outport  Port=3
  wires:
  Sum1/1 -> Fres/1, Divide/1  "Fres"
  Strahl formula/1 -> Gravity/1
  Abs/1 -> Strahl formula/1
  Gravity/1 -> Product/2
  Product/1 -> Sum1/2  "Fw"
  Integrator/1 -> filter out negative velocity/1, Abs/1  "v"
  Constant/1 -> Product/1, Divide/2
  Divide/1 -> Integrator/1  "a"
  p_BP/1 -> Gain/1, Transport Delay/1
  Gain/1 -> Saturation/1
  Gain1/1 -> Sum1/1
  Saturation/1 -> Rate Limiter/1
  Rate Limiter/1 -> Gain1/1
  Transport Delay/1 -> Transfer Fcn/1
  Transfer Fcn/1 -> p_BP_out/1
  filter out negative velocity/1 -> "v "/1

== system Simulation/Subsystem13/Wagon model2 ==
  p_BP : Inport
  Abs : Abs
  Constant : Constant  Value=m
  Divide : Product  Inputs=*/
  Gain : Gain  Gain=-1/(RBD-VBD)
  Gain1 : Gain  Gain=Fb
  Gravity : Gain  Gain=9.81
  Integrator : Integrator  InitialCondition=v0
  Product : Product
  Rate Limiter : RateLimiter  RisingSlewLimit=1/tf  FallingSlewLimit=-1/tl  SampleTimeMode=inherited
  Saturation : Saturate  UpperLimit=1  LowerLimit=0
  Strahl formula : Polyval  Coefs=Pres
  Sum1 : Sum  Inputs=|+-
  Transfer Fcn : TransferFcn  Numerator=BPnum  Denominator=BPden
  Transport Delay : TransportDelay  DelayTime=l/c  InitialOutput=p0
  filter out negative velocity : Saturate  UpperLimit=inf  LowerLimit=0
  Fres : Outport  VectorParamsAs1DForOutWhenUnconnected=off
  p_BP_out : Outport  Port=2  VectorParamsAs1DForOutWhenUnconnected=off
  "v " : Outport  Port=3
  wires:
  Sum1/1 -> Fres/1, Divide/1  "Fres"
  Strahl formula/1 -> Gravity/1
  Abs/1 -> Strahl formula/1
  Gravity/1 -> Product/2
  Product/1 -> Sum1/2  "Fw"
  Constant/1 -> Product/1, Divide/2
  Divide/1 -> Integrator/1  "a"
  p_BP/1 -> Gain/1, Transport Delay/1
  Gain/1 -> Saturation/1
  Gain1/1 -> Sum1/1
  Saturation/1 -> Rate Limiter/1
  Rate Limiter/1 -> Gain1/1
  Transport Delay/1 -> Transfer Fcn/1
  Transfer Fcn/1 -> p_BP_out/1
  Integrator/1 -> filter out negative velocity/1, Abs/1  "v"
  filter out negative velocity/1 -> "v "/1

== system Simulation/Subsystem13/Wagon model3 ==
  p_BP : Inport
  Abs : Abs
  Constant : Constant  Value=m
  Divide : Product  Inputs=*/
  Gain : Gain  Gain=-1/(RBD-VBD)
  Gain1 : Gain  Gain=Fb
  Gravity : Gain  Gain=9.81
  Integrator : Integrator  InitialCondition=v0
  Product : Product
  Rate Limiter : RateLimiter  RisingSlewLimit=1/tf  FallingSlewLimit=-1/tl  SampleTimeMode=inherited
  Saturation : Saturate  UpperLimit=1  LowerLimit=0
  Strahl formula : Polyval  Coefs=Pres
  Sum1 : Sum  Inputs=|+-
  Transfer Fcn : TransferFcn  Numerator=BPnum  Denominator=BPden
  Transport Delay : TransportDelay  DelayTime=l/c  InitialOutput=p0
  filter out negative velocity : Saturate  UpperLimit=inf  LowerLimit=0
  Fres : Outport  VectorParamsAs1DForOutWhenUnconnected=off
  p_BP_out : Outport  Port=2  VectorParamsAs1DForOutWhenUnconnected=off
  "v " : Outport  Port=3
  wires:
  Sum1/1 -> Fres/1, Divide/1  "Fres"
  Strahl formula/1 -> Gravity/1
  Abs/1 -> Strahl formula/1
  Gravity/1 -> Product/2
  Product/1 -> Sum1/2  "Fw"
  Constant/1 -> Product/1, Divide/2
  Divide/1 -> Integrator/1  "a"
  p_BP/1 -> Gain/1, Transport Delay/1
  Gain/1 -> Saturation/1
  Gain1/1 -> Sum1/1
  Saturation/1 -> Rate Limiter/1
  Rate Limiter/1 -> Gain1/1
  Transport Delay/1 -> Transfer Fcn/1
  Transfer Fcn/1 -> p_BP_out/1
  Integrator/1 -> Abs/1, filter out negative velocity/1  "v"
  filter out negative velocity/1 -> "v "/1

== system Simulation/Subsystem13/Wagon model4 ==
  p_BP : Inport
  Abs : Abs
  Constant : Constant  Value=m
  Divide : Product  Inputs=*/
  Gain : Gain  Gain=-1/(RBD-VBD)
  Gain1 : Gain  Gain=Fb
  Gravity : Gain  Gain=9.81
  Integrator : Integrator  InitialCondition=v0
  Product : Product
  Rate Limiter : RateLimiter  RisingSlewLimit=1/tf  FallingSlewLimit=-1/tl  SampleTimeMode=inherited
  Saturation : Saturate  UpperLimit=1  LowerLimit=0
  Strahl formula : Polyval  Coefs=Pres
  Sum1 : Sum  Inputs=|+-
  Transfer Fcn : TransferFcn  Numerator=BPnum  Denominator=BPden
  Transport Delay : TransportDelay  DelayTime=l/c  InitialOutput=p0
  filter out negative velocity : Saturate  UpperLimit=inf  LowerLimit=0
  Fres : Outport  VectorParamsAs1DForOutWhenUnconnected=off
  p_BP_out : Outport  Port=2  VectorParamsAs1DForOutWhenUnconnected=off
  "v " : Outport  Port=3
  wires:
  Sum1/1 -> Fres/1, Divide/1  "Fres"
  Strahl formula/1 -> Gravity/1
  Abs/1 -> Strahl formula/1
  Gravity/1 -> Product/2
  Product/1 -> Sum1/2  "Fw"
  Integrator/1 -> filter out negative velocity/1, Abs/1  "v"
  Constant/1 -> Product/1, Divide/2
  Divide/1 -> Integrator/1  "a"
  p_BP/1 -> Gain/1, Transport Delay/1
  Gain/1 -> Saturation/1
  Gain1/1 -> Sum1/1
  Saturation/1 -> Rate Limiter/1
  Rate Limiter/1 -> Gain1/1
  Transfer Fcn/1 -> p_BP_out/1
  Transport Delay/1 -> Transfer Fcn/1
  filter out negative velocity/1 -> "v "/1

== system Simulation/Subsystem14/Wagon model ==
  note: F = m * a
      | a = F / m
  p_BP : Inport
  Abs : Abs
  Constant : Constant  Value=m
  Divide : Product  Inputs=*/
  Gain : Gain  Gain=-1/(RBD-VBD)
  Gain1 : Gain  Gain=Fb
  Gravity : Gain  Gain=9.81
  Product : Product
  Rate Limiter : RateLimiter  RisingSlewLimit=1/tf  FallingSlewLimit=-1/tl  SampleTimeMode=inherited
  Saturation : Saturate  UpperLimit=1  LowerLimit=0
  Strahl formula : Polyval  Coefs=Pres
  Sum1 : Sum  Inputs=|+-
  Transfer Fcn : TransferFcn  Numerator=BPnum  Denominator=BPden
  Transport Delay : TransportDelay  DelayTime=l/c  InitialOutput=p0
  filter out negative velocity : Saturate  UpperLimit=inf  LowerLimit=0
  v = v0 + a * t : Integrator  InitialCondition=v0
  Fres : Outport  VectorParamsAs1DForOutWhenUnconnected=off
  p_BP_out : Outport  Port=2  VectorParamsAs1DForOutWhenUnconnected=off
  "v " : Outport  Port=3
  wires:
  Sum1/1 -> Fres/1, Divide/1  "Fres"
  Strahl formula/1 -> Gravity/1
  Abs/1 -> Strahl formula/1
  Gravity/1 -> Product/2
  Product/1 -> Sum1/2  "Fw"
  v = v0 + a * t/1 -> filter out negative velocity/1, Abs/1  "v"
  Constant/1 -> Product/1, Divide/2
  Divide/1 -> v = v0 + a * t/1  "a"
  p_BP/1 -> Transport Delay/1, Gain/1
  Gain/1 -> Saturation/1
  Gain1/1 -> Sum1/1
  Saturation/1 -> Rate Limiter/1
  Rate Limiter/1 -> Gain1/1
  Transfer Fcn/1 -> p_BP_out/1
  Transport Delay/1 -> Transfer Fcn/1
  filter out negative velocity/1 -> "v "/1

== system Simulation/Subsystem14/Wagon model1 ==
  p_BP : Inport
  Abs : Abs
  Constant : Constant  Value=m
  Divide : Product  Inputs=*/
  Gain : Gain  Gain=-1/(RBD-VBD)
  Gain1 : Gain  Gain=Fb
  Gravity : Gain  Gain=9.81
  Integrator : Integrator  InitialCondition=v0
  Product : Product
  Rate Limiter : RateLimiter  RisingSlewLimit=1/tf  FallingSlewLimit=-1/tl  SampleTimeMode=inherited
  Saturation : Saturate  UpperLimit=1  LowerLimit=0
  Strahl formula : Polyval  Coefs=Pres
  Sum1 : Sum  Inputs=|+-
  Transfer Fcn : TransferFcn  Numerator=BPnum  Denominator=BPden
  Transport Delay : TransportDelay  DelayTime=l/c  InitialOutput=p0
  filter out negative velocity : Saturate  UpperLimit=inf  LowerLimit=0
  Fres : Outport  VectorParamsAs1DForOutWhenUnconnected=off
  p_BP_out : Outport  Port=2  VectorParamsAs1DForOutWhenUnconnected=off
  "v " : Outport  Port=3
  wires:
  Sum1/1 -> Fres/1, Divide/1  "Fres"
  Strahl formula/1 -> Gravity/1
  Abs/1 -> Strahl formula/1
  Gravity/1 -> Product/2
  Product/1 -> Sum1/2  "Fw"
  Integrator/1 -> filter out negative velocity/1, Abs/1  "v"
  Constant/1 -> Product/1, Divide/2
  Divide/1 -> Integrator/1  "a"
  p_BP/1 -> Gain/1, Transport Delay/1
  Gain/1 -> Saturation/1
  Gain1/1 -> Sum1/1
  Saturation/1 -> Rate Limiter/1
  Rate Limiter/1 -> Gain1/1
  Transport Delay/1 -> Transfer Fcn/1
  Transfer Fcn/1 -> p_BP_out/1
  filter out negative velocity/1 -> "v "/1

== system Simulation/Subsystem14/Wagon model2 ==
  p_BP : Inport
  Abs : Abs
  Constant : Constant  Value=m
  Divide : Product  Inputs=*/
  Gain : Gain  Gain=-1/(RBD-VBD)
  Gain1 : Gain  Gain=Fb
  Gravity : Gain  Gain=9.81
  Integrator : Integrator  InitialCondition=v0
  Product : Product
  Rate Limiter : RateLimiter  RisingSlewLimit=1/tf  FallingSlewLimit=-1/tl  SampleTimeMode=inherited
  Saturation : Saturate  UpperLimit=1  LowerLimit=0
  Strahl formula : Polyval  Coefs=Pres
  Sum1 : Sum  Inputs=|+-
  Transfer Fcn : TransferFcn  Numerator=BPnum  Denominator=BPden
  Transport Delay : TransportDelay  DelayTime=l/c  InitialOutput=p0
  filter out negative velocity : Saturate  UpperLimit=inf  LowerLimit=0
  Fres : Outport  VectorParamsAs1DForOutWhenUnconnected=off
  p_BP_out : Outport  Port=2  VectorParamsAs1DForOutWhenUnconnected=off
  "v " : Outport  Port=3
  wires:
  Sum1/1 -> Fres/1, Divide/1  "Fres"
  Strahl formula/1 -> Gravity/1
  Abs/1 -> Strahl formula/1
  Gravity/1 -> Product/2
  Product/1 -> Sum1/2  "Fw"
  Constant/1 -> Product/1, Divide/2
  Divide/1 -> Integrator/1  "a"
  p_BP/1 -> Gain/1, Transport Delay/1
  Gain/1 -> Saturation/1
  Gain1/1 -> Sum1/1
  Saturation/1 -> Rate Limiter/1
  Rate Limiter/1 -> Gain1/1
  Transport Delay/1 -> Transfer Fcn/1
  Transfer Fcn/1 -> p_BP_out/1
  Integrator/1 -> filter out negative velocity/1, Abs/1  "v"
  filter out negative velocity/1 -> "v "/1

== system Simulation/Subsystem14/Wagon model3 ==
  p_BP : Inport
  Abs : Abs
  Constant : Constant  Value=m
  Divide : Product  Inputs=*/
  Gain : Gain  Gain=-1/(RBD-VBD)
  Gain1 : Gain  Gain=Fb
  Gravity : Gain  Gain=9.81
  Integrator : Integrator  InitialCondition=v0
  Product : Product
  Rate Limiter : RateLimiter  RisingSlewLimit=1/tf  FallingSlewLimit=-1/tl  SampleTimeMode=inherited
  Saturation : Saturate  UpperLimit=1  LowerLimit=0
  Strahl formula : Polyval  Coefs=Pres
  Sum1 : Sum  Inputs=|+-
  Transfer Fcn : TransferFcn  Numerator=BPnum  Denominator=BPden
  Transport Delay : TransportDelay  DelayTime=l/c  InitialOutput=p0
  filter out negative velocity : Saturate  UpperLimit=inf  LowerLimit=0
  Fres : Outport  VectorParamsAs1DForOutWhenUnconnected=off
  p_BP_out : Outport  Port=2  VectorParamsAs1DForOutWhenUnconnected=off
  "v " : Outport  Port=3
  wires:
  Sum1/1 -> Fres/1, Divide/1  "Fres"
  Strahl formula/1 -> Gravity/1
  Abs/1 -> Strahl formula/1
  Gravity/1 -> Product/2
  Product/1 -> Sum1/2  "Fw"
  Constant/1 -> Product/1, Divide/2
  Divide/1 -> Integrator/1  "a"
  p_BP/1 -> Gain/1, Transport Delay/1
  Gain/1 -> Saturation/1
  Gain1/1 -> Sum1/1
  Saturation/1 -> Rate Limiter/1
  Rate Limiter/1 -> Gain1/1
  Transport Delay/1 -> Transfer Fcn/1
  Transfer Fcn/1 -> p_BP_out/1
  Integrator/1 -> Abs/1, filter out negative velocity/1  "v"
  filter out negative velocity/1 -> "v "/1

== system Simulation/Subsystem14/Wagon model4 ==
  p_BP : Inport
  Abs : Abs
  Constant : Constant  Value=m
  Divide : Product  Inputs=*/
  Gain : Gain  Gain=-1/(RBD-VBD)
  Gain1 : Gain  Gain=Fb
  Gravity : Gain  Gain=9.81
  Integrator : Integrator  InitialCondition=v0
  Product : Product
  Rate Limiter : RateLimiter  RisingSlewLimit=1/tf  FallingSlewLimit=-1/tl  SampleTimeMode=inherited
  Saturation : Saturate  UpperLimit=1  LowerLimit=0
  Strahl formula : Polyval  Coefs=Pres
  Sum1 : Sum  Inputs=|+-
  Transfer Fcn : TransferFcn  Numerator=BPnum  Denominator=BPden
  Transport Delay : TransportDelay  DelayTime=l/c  InitialOutput=p0
  filter out negative velocity : Saturate  UpperLimit=inf  LowerLimit=0
  Fres : Outport  VectorParamsAs1DForOutWhenUnconnected=off
  p_BP_out : Outport  Port=2  VectorParamsAs1DForOutWhenUnconnected=off
  "v " : Outport  Port=3
  wires:
  Sum1/1 -> Fres/1, Divide/1  "Fres"
  Strahl formula/1 -> Gravity/1
  Abs/1 -> Strahl formula/1
  Gravity/1 -> Product/2
  Product/1 -> Sum1/2  "Fw"
  Integrator/1 -> filter out negative velocity/1, Abs/1  "v"
  Constant/1 -> Product/1, Divide/2
  Divide/1 -> Integrator/1  "a"
  p_BP/1 -> Gain/1, Transport Delay/1
  Gain/1 -> Saturation/1
  Gain1/1 -> Sum1/1
  Saturation/1 -> Rate Limiter/1
  Rate Limiter/1 -> Gain1/1
  Transfer Fcn/1 -> p_BP_out/1
  Transport Delay/1 -> Transfer Fcn/1
  filter out negative velocity/1 -> "v "/1

== system Simulation/Subsystem15/Wagon model ==
  note: F = m * a
      | a = F / m
  p_BP : Inport
  Abs : Abs
  Constant : Constant  Value=m
  Divide : Product  Inputs=*/
  Gain : Gain  Gain=-1/(RBD-VBD)
  Gain1 : Gain  Gain=Fb
  Gravity : Gain  Gain=9.81
  Product : Product
  Rate Limiter : RateLimiter  RisingSlewLimit=1/tf  FallingSlewLimit=-1/tl  SampleTimeMode=inherited
  Saturation : Saturate  UpperLimit=1  LowerLimit=0
  Strahl formula : Polyval  Coefs=Pres
  Sum1 : Sum  Inputs=|+-
  Transfer Fcn : TransferFcn  Numerator=BPnum  Denominator=BPden
  Transport Delay : TransportDelay  DelayTime=l/c  InitialOutput=p0
  filter out negative velocity : Saturate  UpperLimit=inf  LowerLimit=0
  v = v0 + a * t : Integrator  InitialCondition=v0
  Fres : Outport  VectorParamsAs1DForOutWhenUnconnected=off
  p_BP_out : Outport  Port=2  VectorParamsAs1DForOutWhenUnconnected=off
  "v " : Outport  Port=3
  wires:
  Sum1/1 -> Fres/1, Divide/1  "Fres"
  Strahl formula/1 -> Gravity/1
  Abs/1 -> Strahl formula/1
  Gravity/1 -> Product/2
  Product/1 -> Sum1/2  "Fw"
  v = v0 + a * t/1 -> filter out negative velocity/1, Abs/1  "v"
  Constant/1 -> Product/1, Divide/2
  Divide/1 -> v = v0 + a * t/1  "a"
  p_BP/1 -> Transport Delay/1, Gain/1
  Gain/1 -> Saturation/1
  Gain1/1 -> Sum1/1
  Saturation/1 -> Rate Limiter/1
  Rate Limiter/1 -> Gain1/1
  Transfer Fcn/1 -> p_BP_out/1
  Transport Delay/1 -> Transfer Fcn/1
  filter out negative velocity/1 -> "v "/1

== system Simulation/Subsystem15/Wagon model1 ==
  p_BP : Inport
  Abs : Abs
  Constant : Constant  Value=m
  Divide : Product  Inputs=*/
  Gain : Gain  Gain=-1/(RBD-VBD)
  Gain1 : Gain  Gain=Fb
  Gravity : Gain  Gain=9.81
  Integrator : Integrator  InitialCondition=v0
  Product : Product
  Rate Limiter : RateLimiter  RisingSlewLimit=1/tf  FallingSlewLimit=-1/tl  SampleTimeMode=inherited
  Saturation : Saturate  UpperLimit=1  LowerLimit=0
  Strahl formula : Polyval  Coefs=Pres
  Sum1 : Sum  Inputs=|+-
  Transfer Fcn : TransferFcn  Numerator=BPnum  Denominator=BPden
  Transport Delay : TransportDelay  DelayTime=l/c  InitialOutput=p0
  filter out negative velocity : Saturate  UpperLimit=inf  LowerLimit=0
  Fres : Outport  VectorParamsAs1DForOutWhenUnconnected=off
  p_BP_out : Outport  Port=2  VectorParamsAs1DForOutWhenUnconnected=off
  "v " : Outport  Port=3
  wires:
  Sum1/1 -> Fres/1, Divide/1  "Fres"
  Strahl formula/1 -> Gravity/1
  Abs/1 -> Strahl formula/1
  Gravity/1 -> Product/2
  Product/1 -> Sum1/2  "Fw"
  Integrator/1 -> filter out negative velocity/1, Abs/1  "v"
  Constant/1 -> Product/1, Divide/2
  Divide/1 -> Integrator/1  "a"
  p_BP/1 -> Gain/1, Transport Delay/1
  Gain/1 -> Saturation/1
  Gain1/1 -> Sum1/1
  Saturation/1 -> Rate Limiter/1
  Rate Limiter/1 -> Gain1/1
  Transport Delay/1 -> Transfer Fcn/1
  Transfer Fcn/1 -> p_BP_out/1
  filter out negative velocity/1 -> "v "/1

== system Simulation/Subsystem15/Wagon model2 ==
  p_BP : Inport
  Abs : Abs
  Constant : Constant  Value=m
  Divide : Product  Inputs=*/
  Gain : Gain  Gain=-1/(RBD-VBD)
  Gain1 : Gain  Gain=Fb
  Gravity : Gain  Gain=9.81
  Integrator : Integrator  InitialCondition=v0
  Product : Product
  Rate Limiter : RateLimiter  RisingSlewLimit=1/tf  FallingSlewLimit=-1/tl  SampleTimeMode=inherited
  Saturation : Saturate  UpperLimit=1  LowerLimit=0
  Strahl formula : Polyval  Coefs=Pres
  Sum1 : Sum  Inputs=|+-
  Transfer Fcn : TransferFcn  Numerator=BPnum  Denominator=BPden
  Transport Delay : TransportDelay  DelayTime=l/c  InitialOutput=p0
  filter out negative velocity : Saturate  UpperLimit=inf  LowerLimit=0
  Fres : Outport  VectorParamsAs1DForOutWhenUnconnected=off
  p_BP_out : Outport  Port=2  VectorParamsAs1DForOutWhenUnconnected=off
  "v " : Outport  Port=3
  wires:
  Sum1/1 -> Fres/1, Divide/1  "Fres"
  Strahl formula/1 -> Gravity/1
  Abs/1 -> Strahl formula/1
  Gravity/1 -> Product/2
  Product/1 -> Sum1/2  "Fw"
  Constant/1 -> Product/1, Divide/2
  Divide/1 -> Integrator/1  "a"
  p_BP/1 -> Gain/1, Transport Delay/1
  Gain/1 -> Saturation/1
  Gain1/1 -> Sum1/1
  Saturation/1 -> Rate Limiter/1
  Rate Limiter/1 -> Gain1/1
  Transport Delay/1 -> Transfer Fcn/1
  Transfer Fcn/1 -> p_BP_out/1
  Integrator/1 -> filter out negative velocity/1, Abs/1  "v"
  filter out negative velocity/1 -> "v "/1
